simulink model "SolarPVMPPT"  (R2024b)
settings: Solver=VariableStepAuto  StartTime=0.0  StopTime=20  RelTol=1e-3
libraries: nesl_utility x10, fl_lib x6, ee_lib x2, batteryecm_lib x1, spspowerguiLib x1
settings Model: Creator=agoya  LastModifiedBy=agoyal1642
settings RTWCC: GPUComputeCapability=3.5

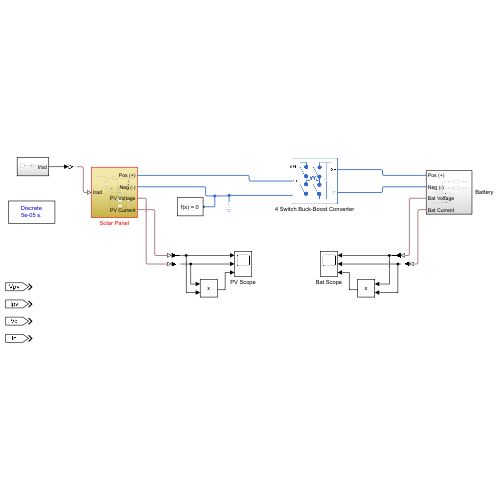
[thumbnail: Simulink's stored preview of the top-level diagram]
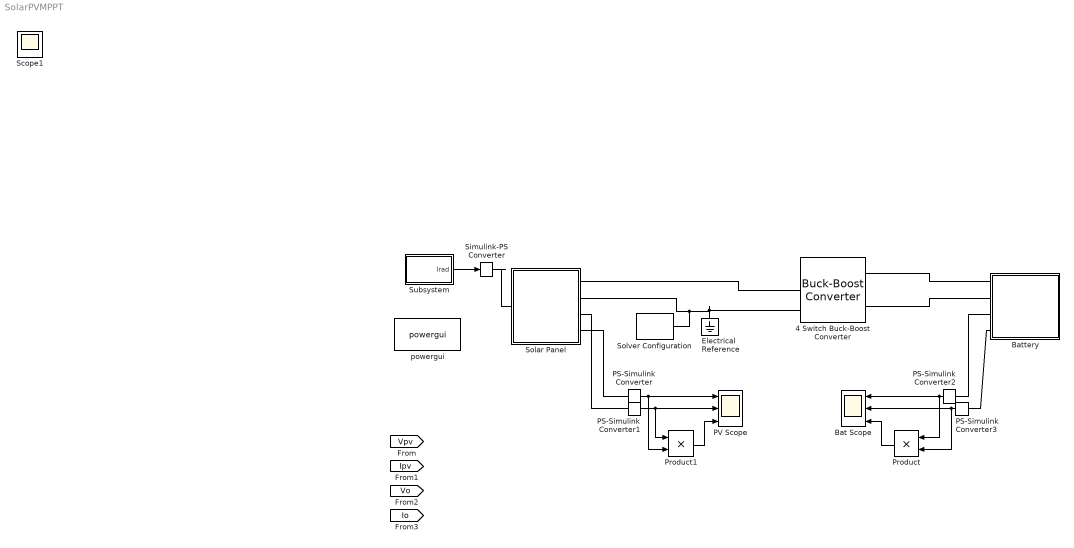
== system SolarPVMPPT ==
  4 Switch Buck-Boost Converter : ee_lib/Semiconductors & Converters/Converters/Buck-Boost Converter  port_option=ee.enum.controlport.ps  device_type=ee.enum.converters.switchingdevice.mosfet  Vf=0.8 V  Ron=0.001 Ohm  Rds=0.001 Ohm  Goff=1e-5 1/Ohm  Vgt=1 V  Vgt_off=-1 V  Ih=1 A  Vth=6 V  K=0  diode_param=ee.enum.converters.diode.nodynamics  diode_Vf=0.8 V  diode_Ron=0.001 Ohm  diode_Goff=1e-5 1/Ohm  diode_C=50 nF  diode_iRM=-235 A  diode_iF=300 A  diode_idot=-50 A/us  diode_trr_param=ee.enum.converters.diodetrr.trr_factor  diode_trr_factor=3  diode_trr=15 us  diode_Qrr=1500 s*uA  Lf=1e-6 H  Rl=0 Ohm  Cf=1e-7 F  Rf=1e-6 Ohm  snubber_type=ee.enum.converters.snubber.exclude  Cs=1e-7 F  Rs=0.1 Ohm  iL_specify=off  iL_priority=High  iL=0 A  iL_nominal_specify=off  iL_nominal_value=1  iL_nominal_unit=A  vc_specify=off  vc_priority=High  vc=0 V  vc_nominal_specify=off  vc_nominal_value=1  vc_nominal_unit=V
      settings: InternalSimscapePortConfiguration="{\"Bottom\":[],\"Left\":[{\"id\":\"G\",\"label\":\"G\",\"type\":\"foundation.electrical.eight_phase\"},{\"id\":\"p1\",\"label\":\"1+\",\"type\":\"foundation.electrical.electrical\"},{\"id\":\"n1\",\"label\":\"1-\",\"type\":\"foundation.electrical.electrical\"}],\"Right\":[{\"id\":\"p2\",\"label\":\"2+\",\"type\":\"foundation.electrical.electrical\"},{\"id\":\"n2\",\"label\":\"2-\",\"type\":\"foundation.electrical.electrical\"}],\"Top\":[]}"
  Bat Scope : Scope  NumInputPorts=3
  Battery : Subsystem
  Electrical Reference : fl_lib/Electrical/Electrical Elements/Electrical Reference
  PS-Simulink Converter{,1..3} (4 alike) : nesl_utility/PS-Simulink Converter  PhysicalDomain=network_engine_domain  SubClassName=ps_output  LeftPortType=input  RightPortType=output  PseudoPeriodic=off  Frequencies=[]  VectorFormat=inherit  Unit=inherit  AffineConversion=off
  PV Scope : Scope  NumInputPorts=3
  Product : Product
  Product1 : Product
  Simulink-PS Converter : nesl_utility/Simulink-PS Converter  PhysicalDomain=network_engine_domain  SubClassName=ps_input  LeftPortType=input  RightPortType=output  PseudoPeriodic=off  Frequencies=[]  NoiseDistribution=none  NoiseParameters=[]  Unit=1  AffineConversion=off  FilteringAndDerivatives=provide  SimscapeFilterOrder=1  InputFilterTimeConstant=0.001  UdotUserProvided=0
  Solar Panel : Subsystem
  Solver Configuration : nesl_utility/Solver Configuration  PhysicalDomain=network_engine_domain  SubClassName=solver  LeftPortType=input  RightPortType=generic  Tones=[]  Harmonics=[]  SimulateNoise=off  Profile=off  UseLocalSampling=off  EnableSwitchedLinearOptims=on  FrequencyDomain=off  UseCCode=off  RelTol=0.001  AbsTol=0.001  MinStep=1e-09  ToWorkspace=off  RevertToSquareIcSolve=off  NumHomotopyIterations=100  PhasorMode=off  PhasorModeNumHarmonics=1  ConsistencySolver=NEWTON_XTOL_AFTER_FTOL  IndexReductionMethod=DerivativeReplacement  DoDC=off  ResidualTolerance=1e-09  ConsistencyTolSource=GLOBAL  ConsistencyAbsTol=0.001  ConsistencyRelTol=0.001  ConsistencyTolFactor=0.001  UseLocalSolver=off  LocalSolverChoice=NE_BACKWARD_EULER_ADVANCER  ResolveIndetEquations=on  FunctionEvalNumThread=1  LocalSolverSampleTime=0.001  DoFixedCost=off  MaxNonlinIter=3  MaxModeIter=2  ComputeImpulses=off  ImpulseIterations=2  LinearAlgebra=auto  LinearAlgebraNumThread=0  EquationFormulation=NE_TIME_EF  DelaysMemoryBudget=1024  AutomaticFiltering=on  FilteringTimeConstant=0.001  PartitionStorageMethod=AS_NEEDED  PartitionMemoryBudget=1024  PartitionMethod=ROBUST  MultibodyUseLocalSolver=off  MultibodyLocalSolverChoice=ODE1  MultibodyLocalSolverSampleTime=0.001
  Subsystem : Subsystem
  powergui : spspowerguiLib/powergui  Priority=1  SimulationMode=Discrete  SampleTime=50e-6  frequency=60  Iterations=50  frequencyindice=0  Pbase=100e6  ErrMax=1e-4  UnitsV=kV  UnitsW=MW  buscounter=0  FunctionMessages=off  echomessages=off  EnableUseOfTLC=off  CurrentSourceSwitches=off  DisableSnubberDevices=off  DisableRonSwitches=off  DisableVfSwitches=off  DisplayEquations=off  AutomaticDiscreteSolvers=off  SolverType=Tustin/Backward Euler (TBE)  Interpol=off  ExternalGateDelay=off  methode=off  Ts=100  x0status=blocks  SPID=on  SwTol=0  HookPort=off  NonlinearTolerance=1e-4  nMaxIteration=100  ContinueOnMaxIteration=off  RestoreLinks=warning  ResistiveCurrentMeasurement=off  Frange=[0:2:500]  Ylog=off  Xlog=on  ShowGrid=off  save=off  variable=ZData  structure=0  ZoomFFT=off  StartTime=0.0  cycles=1  DisplayStyle=1  fundamental=60  FreqAxis=off  MaxFrequency=1000  frequencyindicesteady=1  RmsSteady=1  display=off
  Scope1 : Scope
  wires:
  Subsystem/1(Irad) -> Simulink-PS Converter/1
  PS-Simulink Converter/1 -> Product1/2, PV Scope/1
  PS-Simulink Converter1/1 -> Product1/1, PV Scope/2
  PS-Simulink Converter3/1 -> Product/2, Bat Scope/2
  PS-Simulink Converter2/1 -> Product/1, Bat Scope/1
  Product/1 -> Bat Scope/3
  Product1/1 -> PV Scope/3
  connections:
  Simulink-PS Converter/RConn1 -- Solar Panel/LConn1
  Solar Panel/RConn2 -- Solver Configuration/RConn1 -- Electrical Reference/LConn1 -- 4 Switch Buck-Boost Converter/LConn3
  4 Switch Buck-Boost Converter/RConn2 -- Battery/LConn2
  Solar Panel/RConn1 -- 4 Switch Buck-Boost Converter/LConn2
  4 Switch Buck-Boost Converter/RConn1 -- Battery/LConn1
  Solar Panel/RConn4 -- PS-Simulink Converter/LConn1
  Solar Panel/RConn3 -- PS-Simulink Converter1/LConn1
  PS-Simulink Converter2/LConn1 -- Battery/LConn3
  PS-Simulink Converter3/LConn1 -- Battery/LConn4

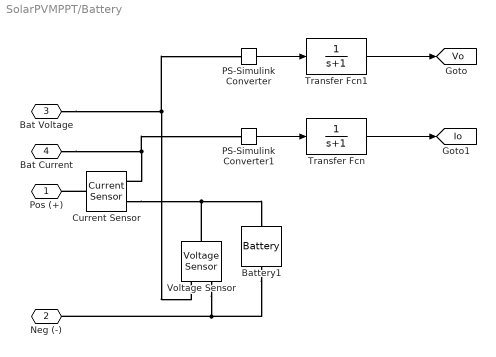
== system SolarPVMPPT/Battery ==
  Battery1 : batteryecm_lib/Battery  Vnom=49 V  prm_dir=simscape.enum.battery.prm_dir.disabled  R1_dis=2 Ohm  R1_ch=2 Ohm  R1=2 Ohm  prm_AH=simscape.enum.battery.prm_AH.infinite  AH=50 A*hr  V1=11.5 V  AH1=25 A*hr  prm_R2=simscape.enum.battery.prm_R2.disabled  R2=2000 Ohm  Tmeas=298.15 K  charge_measurement_port=simscape.enum.battery.enable.no  prm_dyn=simscape.enum.battery.prm_dyn.off  Rp1=0.005 Ohm  tau1=30 s  Rp2=0.005 Ohm  tau2=30 s  Rp3=0.005 Ohm  tau3=30 s  Rp4=0.005 Ohm  tau4=30 s  Rp5=0.005 Ohm  tau5=30 s  prm_fade=simscape.enum.battery.prm_fade.disabled  N_fade=100  AH_fade=45 A*hr  R1_fade=2.02 Ohm  R1_ch_fade=2.02 Ohm  V1_fade=10.35 V  prm_age=simscape.enum.battery.prm_age.disabled  prm_age_OCV=simscape.enum.battery.prm_age_OCV.OCV  OCV_age=0.9  SOC_age=60  Tmeas_age=298.15 K  delta_time_age_vec=[0] d  temperature_age_vec=[273] K  OCV_scaling_age=2.2134e6  OCV_offset_age=1.632e6  temp_exp_age=0.515833569 V  t_exp_age=0.75  Vnom_T2=12 V  R1_T2=2.2 Ohm  R1_T2_dis=2.2 Ohm  R1_T2_ch=2.2 Ohm  V1_T2=11.4 V  R2_T2=2200 Ohm  Rp1_T2=0.005 Ohm  tau1_T2=30 s  Rp2_T2=0.005 Ohm  tau2_T2=30 s  Rp3_T2=0.005 Ohm  tau3_T2=30 s  Rp4_T2=0.005 Ohm  tau4_T2=30 s  Rp5_T2=0.005 Ohm  tau5_T2=30 s  Tmeas2=273.15 K  thermal_port=simscape.enum.thermaleffects.omit  thermal_mass=30000 J/K  i_specify=off  i_priority=None  i=0 A  i_nominal_specify=off  i_nominal_value=1  i_nominal_unit=A  v_specify=off  v_priority=None  v=0 V  v_nominal_specify=off  v_nominal_value=1  v_nominal_unit=V  charge_specify=off  charge_priority=High  charge=50 A*hr  charge_nominal_specify=off  charge_nominal_value=1  charge_nominal_unit=A*hr  num_cycles_specify=off  num_cycles_priority=High  num_cycles=0  num_cycles_nominal_specify=off  num_cycles_nominal_value=1  num_cycles_nominal_unit=1  temperature_specify=off  temperature_priority=High  temperature=298.15 K  temperature_nominal_specify=off  temperature_nominal_value=1  temperature_nominal_unit=K
  Current Sensor : fl_lib/Electrical/Electrical Sensors/Current Sensor
  PS-Simulink Converter : nesl_utility/PS-Simulink Converter  PhysicalDomain=network_engine_domain  SubClassName=ps_output  LeftPortType=input  RightPortType=output  PseudoPeriodic=off  Frequencies=[]  VectorFormat=inherit  Unit=inherit  AffineConversion=off
  PS-Simulink Converter1 : nesl_utility/PS-Simulink Converter  PhysicalDomain=network_engine_domain  SubClassName=ps_output  LeftPortType=input  RightPortType=output  PseudoPeriodic=off  Frequencies=[]  VectorFormat=inherit  Unit=inherit  AffineConversion=off
  Transfer Fcn : TransferFcn  Denominator=[1 1]
  Transfer Fcn1 : TransferFcn  Denominator=[1 1]
  Voltage Sensor : fl_lib/Electrical/Electrical Sensors/Voltage Sensor
  Pos (+) : PMIOPort  Side=Left
  Neg (-) : PMIOPort  Port=2  Side=Left
  Bat Voltage : PMIOPort  Port=3  Side=Left
  Bat Current : PMIOPort  Port=4  Side=Left
  tag scope: Io=global, Vo=global
  wires:
  PS-Simulink Converter/1 -> Transfer Fcn1/1
  PS-Simulink Converter1/1 -> Transfer Fcn/1
  Transfer Fcn/1 -> [Io]
  Transfer Fcn1/1 -> [Vo]
  connections:
  Battery1/RConn1 -- Neg (-)/RConn1 -- Voltage Sensor/RConn2
  Current Sensor/LConn1 -- Pos (+)/RConn1
  Current Sensor/RConn2 -- Battery1/LConn1 -- Voltage Sensor/LConn1
  Bat Voltage/RConn1 -- PS-Simulink Converter/LConn1 -- Voltage Sensor/RConn1
  Bat Current/RConn1 -- PS-Simulink Converter1/LConn1 -- Current Sensor/RConn1

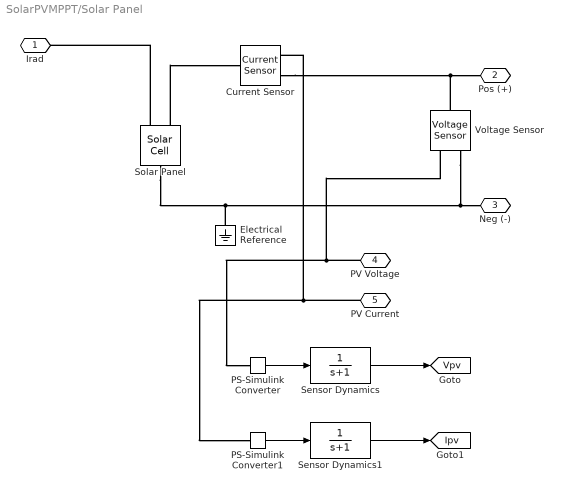
== system SolarPVMPPT/Solar Panel ==
  Current Sensor : fl_lib/Electrical/Electrical Sensors/Current Sensor
  Electrical Reference : fl_lib/Electrical/Electrical Elements/Electrical Reference
  PS-Simulink Converter : nesl_utility/PS-Simulink Converter  PhysicalDomain=network_engine_domain  SubClassName=ps_output  LeftPortType=input  RightPortType=output  PseudoPeriodic=off  Frequencies=[]  VectorFormat=inherit  Unit=inherit  AffineConversion=off
  PS-Simulink Converter1 : nesl_utility/PS-Simulink Converter  PhysicalDomain=network_engine_domain  SubClassName=ps_output  LeftPortType=input  RightPortType=output  PseudoPeriodic=off  Frequencies=[]  VectorFormat=inherit  Unit=inherit  AffineConversion=off
  Sensor Dynamics : TransferFcn  Denominator=[1 1]
  Sensor Dynamics1 : TransferFcn  Denominator=[1 1]
  Solar Panel : ee_lib/Sources/Solar Cell  PartSpecification="{\"DatasetId\":\"Hanwha_Q_CELLS|QPEAK_DUO_L_G5_400|simscape.electrical.solarCell\",\"DisplayName\":\"Hanwha_Q_CELLS:QPEAK_DUO_L_G5_400\"}"  prm=ee.enum.sources.solar_cell_prm.datasheet  Isc=5.1442 A  Voc=0.6814 V  Is=1.1034286341295e-07 A  Is2=6.11780423347103e-10 A  Iph=5.14424134114276 A  Ir0=1000 W/m^2  ec=1.50197733551845  N2=1.39390149326833  Rs=3.58542098290393e-07 Ohm  Rp=1667.59911707245 Ohm  N_series=72  N_parallel=2  TIPH1=0.00028030217063849 1/K  EG=1.12 eV  TXIS1=3.81507066256415  TXIS2=12.2423010919844  TRS1=0.309203055876839  TRP1=0 % Parameter not set  Tmeas=25 degC  TFIXED=25 degC  thermal_mass=100 % Parameter not set J/K  initial_temperature=25 degC
      settings: AttributesFormatString=Hanwha_Q_CELLS:QPEAK_DUO_L_G5_400
  Voltage Sensor : fl_lib/Electrical/Electrical Sensors/Voltage Sensor
  Irad : PMIOPort  Side=Left
  Pos (+) : PMIOPort  Port=2  Side=Right
  Neg (-) : PMIOPort  Port=3  Side=Right
  PV Voltage : PMIOPort  Port=4  Side=Right
  PV Current : PMIOPort  Port=5  Side=Right
  tag scope: Ipv=global, Vpv=global
  wires:
  PS-Simulink Converter/1 -> Sensor Dynamics/1
  Sensor Dynamics/1 -> [Vpv]
  Sensor Dynamics1/1 -> [Ipv]
  PS-Simulink Converter1/1 -> Sensor Dynamics1/1
  connections:
  Solar Panel/RConn1 -- Electrical Reference/LConn1 -- Voltage Sensor/RConn2 -- Neg (-)/RConn1
  Solar Panel/LConn1 -- Irad/RConn1
  Solar Panel/LConn2 -- Current Sensor/LConn1
  Current Sensor/RConn2 -- Voltage Sensor/LConn1 -- Pos (+)/RConn1
  PV Current/RConn1 -- PS-Simulink Converter1/LConn1 -- Current Sensor/RConn1
  PV Voltage/RConn1 -- PS-Simulink Converter/LConn1 -- Voltage Sensor/RConn1

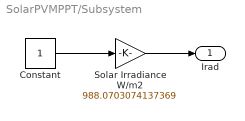
== system SolarPVMPPT/Subsystem ==
  Constant : Constant
  Solar Irradiance W/m2 : Gain  Gain=988.0703074137369
  Irad : Outport
  wires:
  Constant/1 -> Solar Irradiance W/m2/1
  Solar Irradiance W/m2/1 -> Irad/1
